simulink model "Caso10EDOLipschitzLocalGlobal"  (R2015a)
settings: Solver=ode45  StartTime=0.0  StopTime=10  FixedStep=0.00001  MaxStep=1e-1  RelTol=1e-3
libraries: simulink x4
settings Model: Creator=user  LastModifiedBy=user
settings SolverCC: ShapePreserveControl=EnableAll  ZeroCrossControl=DisableAll

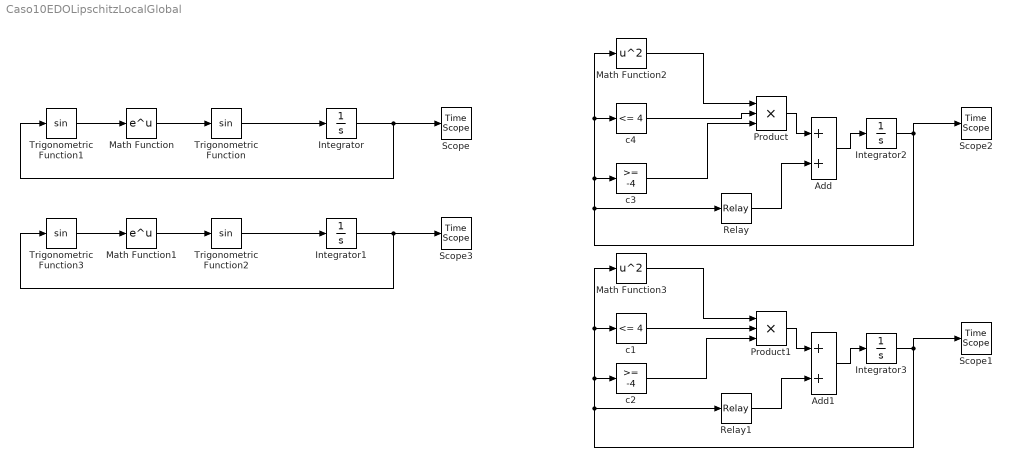
== system Caso10EDOLipschitzLocalGlobal ==
  Add : Sum
  Add1 : Sum
  Integrator : Integrator  InitialCondition=-1000
  Integrator1 : Integrator
  Integrator2 : Integrator  InitialCondition=1
  Integrator3 : Integrator  InitialCondition=50
  Math Function : Math  SaturateOnIntegerOverflow=on
  Math Function1 : Math  SaturateOnIntegerOverflow=on
  Math Function2 : Math  Operator=square  SaturateOnIntegerOverflow=on
  Math Function3 : Math  Operator=square  SaturateOnIntegerOverflow=on
  Product : Product  Inputs=3
  Product1 : Product  Inputs=3
  Relay : Relay  OnSwitchValue=4  OffSwitchValue=4  OnOutputValue=-4
  Relay1 : Relay  OnSwitchValue=4  OffSwitchValue=4  OnOutputValue=-4
  Scope{,1..3} (4 alike) : TimeScope
  Trigonometric Function{,1..3} (4 alike) : Trigonometry
  c1 : simulink/Logic and Bit Operations/Compare To Constant  relop=<=  const=4  OutDataTypeStr=boolean
  c2 : simulink/Logic and Bit Operations/Compare To Constant  relop=>=  const=-4  OutDataTypeStr=boolean
  c3 : simulink/Logic and Bit Operations/Compare To Constant  relop=>=  const=-4  OutDataTypeStr=boolean
  c4 : simulink/Logic and Bit Operations/Compare To Constant  relop=<=  const=4  OutDataTypeStr=boolean
  wires:
  Math Function/1 -> Trigonometric Function/1
  Trigonometric Function1/1 -> Math Function/1
  Integrator/1 -> Trigonometric Function1/1, Scope/1
  Trigonometric Function/1 -> Integrator/1
  Math Function1/1 -> Trigonometric Function2/1
  Trigonometric Function3/1 -> Math Function1/1
  Integrator1/1 -> Scope3/1, Trigonometric Function3/1
  Trigonometric Function2/1 -> Integrator1/1
  Product/1 -> Add/1
  Add/1 -> Integrator2/1
  Relay/1 -> Add/2
  Integrator2/1 -> Scope2/1, Math Function2/1, c4/1, c3/1, Relay/1
  c4/1 -> Product/2
  Product1/1 -> Add1/1
  Add1/1 -> Integrator3/1
  Relay1/1 -> Add1/2
  Integrator3/1 -> Scope1/1, c2/1, Math Function3/1, c1/1, Relay1/1
  c1/1 -> Product1/2
  Math Function2/1 -> Product/1
  Math Function3/1 -> Product1/1
  c2/1 -> Product1/3
  c3/1 -> Product/3
